simulink model "test_resync_new"  (Simulink 7.4)
settings: Solver=ode45  StartTime=0  StopTime=300  RelTol=1e-3
libraries: xbsIndex_r4 x37, casper_library x1, xps_library x1
settings Model: Creator=wjm  LastModifiedBy=wjm
settings OptimizationCC: InitFltsAndDblsToZero=on

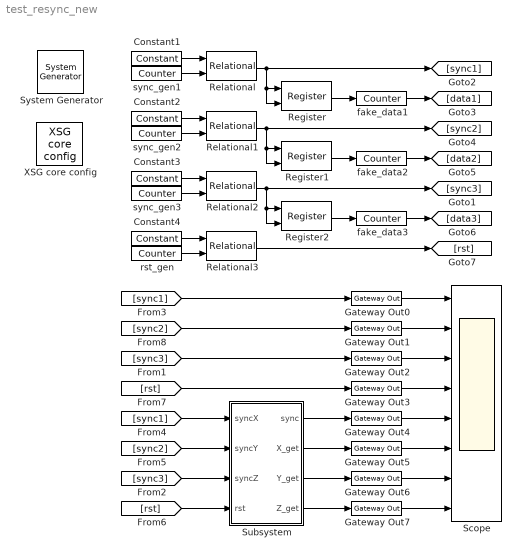
== system test_resync_new ==
  " System Generator" : xbsIndex_r4/ System Generator  Tag=genX  SystemSampleTime=-1  xilinxfamily=virtex5  part=xc5vsx95t  speed=-1  package=ff1136  synthesis_tool=XST  clock_wrapper=Clock Enables  directory=./isi_correlator_cropped/sysgen  testbench=off  simulink_period=1  sysclk_period=5  dcm_input_clock_period=100  incr_netlist=off  trim_vbits=Everywhere in SubSystem  dbl_ovrd=According to Block Masks  core_generation=According to Block Masks  run_coregen=off  deprecated_control=off  eval_field=0  block_type=sysgen
      settings: block_version=10.1.1
  Constant1 : xbsIndex_r4/Constant  arith_type=Unsigned  const=10  n_bits=7  bin_pt=0  explicit_period=on  period=1  equ=P=C  opselect=C  inp2=PCIN>>17  opr=+  inp1=P  carry=CIN  dbl_ovrd=off  block_type=constant
  Constant2 : xbsIndex_r4/Constant  arith_type=Unsigned  const=15  n_bits=7  bin_pt=0  explicit_period=on  period=1  equ=P=C  opselect=C  inp2=PCIN>>17  opr=+  inp1=P  carry=CIN  dbl_ovrd=off  block_type=constant
  Constant3 : xbsIndex_r4/Constant  arith_type=Unsigned  const=20  n_bits=7  bin_pt=0  explicit_period=on  period=1  equ=P=C  opselect=C  inp2=PCIN>>17  opr=+  inp1=P  carry=CIN  dbl_ovrd=off  block_type=constant
  Constant4 : xbsIndex_r4/Constant  arith_type=Unsigned  const=5  n_bits=8  bin_pt=0  explicit_period=on  period=1  equ=P=C  opselect=C  inp2=PCIN>>17  opr=+  inp1=P  carry=CIN  dbl_ovrd=off  block_type=constant
  Gateway Out{0..7} (8 alike) : xbsIndex_r4/Gateway Out  hdl_port=on  timing_constraint=None  locs_specified=off  LOCs={}  block_type=gatewayout
      settings: infoedit="Gateway out block.  Converts Xilinx fixed point inputs into ouputs of type Simulink integer, double, or fixed point.<br><br>Hardware notes:  In hardware these blocks become top level output ports or are discarded, depending on how they are configured."  block_version=11.3
  Register : xbsIndex_r4/Register  init=0  rst=off  en=on  dbl_ovrd=off  block_type=register
  Register1 : xbsIndex_r4/Register  init=0  rst=off  en=on  dbl_ovrd=off  block_type=register
  Register2 : xbsIndex_r4/Register  init=0  rst=off  en=on  dbl_ovrd=off  block_type=register
  Relational{,1..3} (4 alike) : xbsIndex_r4/Relational  mode=a=b  en=off  latency=1  dbl_ovrd=off  block_type=relational
  Scope : Scope  NumInputPorts=8
      settings: YMin=0~0~0~0~0~0~0~-5  YMax=1~35~1~35~1~35~1~5
  Subsystem : Subsystem
  XSG core config : xps_library/XSG core config  Tag=xps:xsg  SystemSampleTime=-1  hw_sys=ROACH:sx95t  ibob_linux=off  clk_src=adc0_clk  iBOB_clk_src=sys_clk  BEE2_ctrl_clk_src=sys_clk  BEE2_usr_clk_src=sys_clk  ROACH_clk_src=adc0_clk  CORR_clk_src=sys_clk  gpio_clk_io_group=iBOB:sma  gpio_clk_bit_index=0  clk_rate=200  sample_period=1  synthesis_tool=XST  mpc_type=powerpc440_ext
  fake_data1 : xbsIndex_r4/Counter  cnt_type=Free Running  cnt_to=Inf  operation=Up  start_count=0  cnt_by_val=1  arith_type=Unsigned  n_bits=5  bin_pt=0  load_pin=off  rst=off  en=on  explicit_period=on  period=1  dbl_ovrd=off  use_behavioral_HDL=off  implementation=Fabric  use_rpm=off  block_type=counter
  fake_data2 : xbsIndex_r4/Counter  cnt_type=Free Running  cnt_to=Inf  operation=Down  start_count=2^5 - 1  cnt_by_val=1  arith_type=Unsigned  n_bits=5  bin_pt=0  load_pin=off  rst=off  en=on  explicit_period=on  period=1  dbl_ovrd=off  use_behavioral_HDL=off  implementation=Fabric  use_rpm=off  block_type=counter
  fake_data3 : xbsIndex_r4/Counter  cnt_type=Free Running  cnt_to=Inf  operation=Down  start_count=2^5 - 1  cnt_by_val=1  arith_type=Unsigned  n_bits=5  bin_pt=0  load_pin=off  rst=off  en=on  explicit_period=on  period=1  dbl_ovrd=off  use_behavioral_HDL=off  implementation=Fabric  use_rpm=off  block_type=counter
  rst_gen : xbsIndex_r4/Counter  cnt_type=Free Running  cnt_to=Inf  operation=Up  start_count=0  cnt_by_val=1  arith_type=Unsigned  n_bits=8  bin_pt=0  load_pin=off  rst=off  en=off  explicit_period=on  period=1  dbl_ovrd=off  use_behavioral_HDL=off  implementation=Fabric  use_rpm=off  block_type=counter
  sync_gen1 : xbsIndex_r4/Counter  cnt_type=Free Running  cnt_to=Inf  operation=Up  start_count=0  cnt_by_val=1  arith_type=Unsigned  n_bits=7  bin_pt=0  load_pin=off  rst=off  en=off  explicit_period=on  period=1  dbl_ovrd=off  use_behavioral_HDL=off  implementation=Fabric  use_rpm=off  block_type=counter
  sync_gen2 : xbsIndex_r4/Counter  cnt_type=Free Running  cnt_to=Inf  operation=Up  start_count=0  cnt_by_val=1  arith_type=Unsigned  n_bits=7  bin_pt=0  load_pin=off  rst=off  en=off  explicit_period=on  period=1  dbl_ovrd=off  use_behavioral_HDL=off  implementation=Fabric  use_rpm=off  block_type=counter
  sync_gen3 : xbsIndex_r4/Counter  cnt_type=Free Running  cnt_to=Inf  operation=Up  start_count=0  cnt_by_val=1  arith_type=Unsigned  n_bits=7  bin_pt=0  load_pin=off  rst=off  en=off  explicit_period=on  period=1  dbl_ovrd=off  use_behavioral_HDL=off  implementation=Fabric  use_rpm=off  block_type=counter
  wires:
  Gateway Out1/1 -> Scope/2
  Gateway Out2/1 -> Scope/3
  Gateway Out3/1 -> Scope/4
  Gateway Out4/1 -> Scope/5
  Constant1/1 -> Relational/1
  sync_gen1/1 -> Relational/2
  Gateway Out0/1 -> Scope/1
  Gateway Out5/1 -> Scope/6
  Gateway Out6/1 -> Scope/7
  Constant2/1 -> Relational1/1
  sync_gen2/1 -> Relational1/2
  Relational/1 -> Register/1, Register/2, [sync1]
  Relational1/1 -> [sync2], Register1/2, Register1/1
  Register1/1 -> fake_data2/1
  fake_data2/1 -> [data2]
  Register/1 -> fake_data1/1
  fake_data1/1 -> [data1]
  Constant3/1 -> Relational2/1
  sync_gen3/1 -> Relational2/2
  Relational2/1 -> [sync3], Register2/2, Register2/1
  Register2/1 -> fake_data3/1
  fake_data3/1 -> [data3]
  [sync1] -> Gateway Out0/1
  [sync2] -> Gateway Out1/1
  [sync3] -> Gateway Out2/1
  [sync1] -> Subsystem/1(syncX)
  [sync2] -> Subsystem/2(syncY)
  [sync3] -> Subsystem/3(syncZ)
  Constant4/1 -> Relational3/1
  rst_gen/1 -> Relational3/2
  Relational3/1 -> [rst]
  [rst] -> Subsystem/4(rst)
  Gateway Out7/1 -> Scope/8
  [rst] -> Gateway Out3/1
  Subsystem/1(sync) -> Gateway Out4/1
  Subsystem/2(X_get) -> Gateway Out5/1
  Subsystem/3(Y_get) -> Gateway Out6/1
  Subsystem/4(Z_get) -> Gateway Out7/1

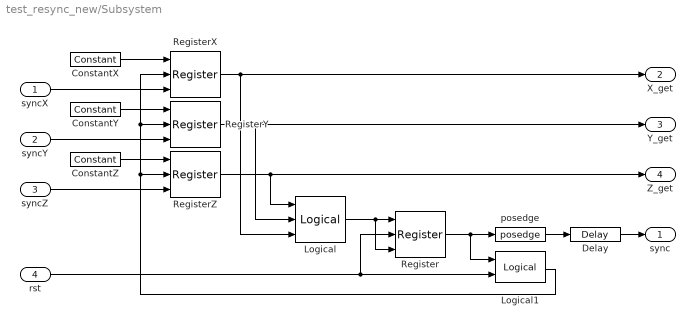
== system test_resync_new/Subsystem ==
  syncX : Inport  OutDataType=sfix(16)  OutScaling=2^0
  syncY : Inport  Port=2  OutDataType=sfix(16)  OutScaling=2^0
  syncZ : Inport  Port=3  OutDataType=sfix(16)  OutScaling=2^0
  rst : Inport  Port=4  OutDataType=sfix(16)  OutScaling=2^0
  ConstantX : xbsIndex_r4/Constant  arith_type=Boolean  const=0  n_bits=1  bin_pt=0  explicit_period=on  period=1  equ=P=C  opselect=C  inp2=PCIN>>17  opr=+  inp1=P  carry=CIN  dbl_ovrd=off  block_type=constant
      settings: block_version=10.1.1
  ConstantY : xbsIndex_r4/Constant  arith_type=Boolean  const=0  n_bits=1  bin_pt=0  explicit_period=on  period=1  equ=P=C  opselect=C  inp2=PCIN>>17  opr=+  inp1=P  carry=CIN  dbl_ovrd=off  block_type=constant
      settings: block_version=10.1.1
  ConstantZ : xbsIndex_r4/Constant  arith_type=Boolean  const=0  n_bits=1  bin_pt=0  explicit_period=on  period=1  equ=P=C  opselect=C  inp2=PCIN>>17  opr=+  inp1=P  carry=CIN  dbl_ovrd=off  block_type=constant
      settings: block_version=10.1.1
  Delay : xbsIndex_r4/Delay  en=off  latency=3  dbl_ovrd=off  reg_retiming=on  block_type=delay
  Logical : xbsIndex_r4/Logical  logical_function=NOR  inputs=3  en=off  latency=1  precision=Full  arith_type=Unsigned  n_bits=16  bin_pt=0  align_bp=on  dbl_ovrd=off  block_type=logical
      settings: block_version=11.4
  Logical1 : xbsIndex_r4/Logical  logical_function=OR  inputs=2  en=off  latency=0  precision=Full  arith_type=Unsigned  n_bits=16  bin_pt=0  align_bp=on  dbl_ovrd=off  block_type=logical
      settings: block_version=11.4
  Register : xbsIndex_r4/Register  init=0  rst=on  en=on  dbl_ovrd=off  block_type=register
      settings: block_version=11.4
  RegisterX : xbsIndex_r4/Register  init=1  rst=on  en=on  dbl_ovrd=off  block_type=register
      settings: block_version=11.4
  RegisterY : xbsIndex_r4/Register  init=1  rst=on  en=on  dbl_ovrd=off  block_type=register
      settings: block_version=11.4
  RegisterZ : xbsIndex_r4/Register  init=1  rst=on  en=on  dbl_ovrd=off  block_type=register
      settings: block_version=11.4
  posedge : casper_library/Misc/posedge  Tag=Rising Edge Detector  SystemSampleTime=-1
  sync : Outport  OutDataType=sfix(16)  OutScaling=2^0
  X_get : Outport  Port=2  OutDataType=sfix(16)  OutScaling=2^0
  Y_get : Outport  Port=3  OutDataType=sfix(16)  OutScaling=2^0
  Z_get : Outport  Port=4  OutDataType=sfix(16)  OutScaling=2^0
  wires:
  ConstantX/1 -> RegisterX/1
  ConstantY/1 -> RegisterY/1
  ConstantZ/1 -> RegisterZ/1
  syncX/1 -> RegisterX/3
  syncY/1 -> RegisterY/3
  syncZ/1 -> RegisterZ/3
  RegisterY/1 -> Y_get/1, Logical/2
  RegisterX/1 -> X_get/1, Logical/3
  RegisterZ/1 -> Z_get/1, Logical/1
  Logical/1 -> Register/1, Register/3
  posedge/1 -> Delay/1
  Delay/1 -> sync/1
  Register/1 -> Logical1/1, posedge/1
  rst/1 -> Logical1/2, Register/2
  Logical1/1 -> RegisterX/2, RegisterY/2, RegisterZ/2
